simulink model "Flyback_non_ideal_simulation0101"  (R2023b)
settings: Solver=VariableStepAuto  StartTime=0.0  StopTime=0.01  RelTol=1e-3
libraries: spsMeanLib x6, spsCurrentMeasurementLib x4, spsMultimeterLib x4, spsSeriesRLCBranchLib x4, spsDiodeLib x3, spsMosfetLib x3, spsDCVoltageSourceLib x2, spsLinearTransformerLib x2, spsRMSLib x2, spsVoltageMeasurementLib x2, sps_lib x1
settings Model: Creator=User  LastModifiedBy=ozgur

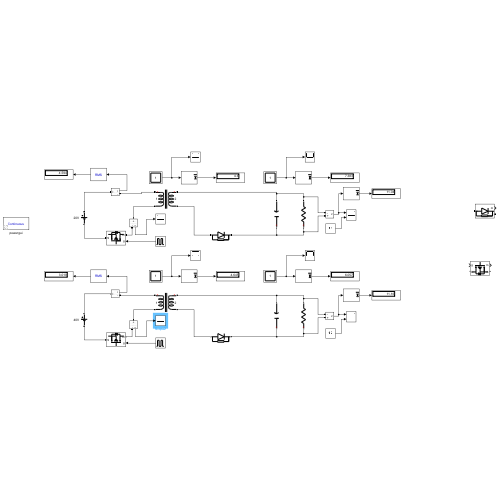
[thumbnail: Simulink's stored preview of the top-level diagram]
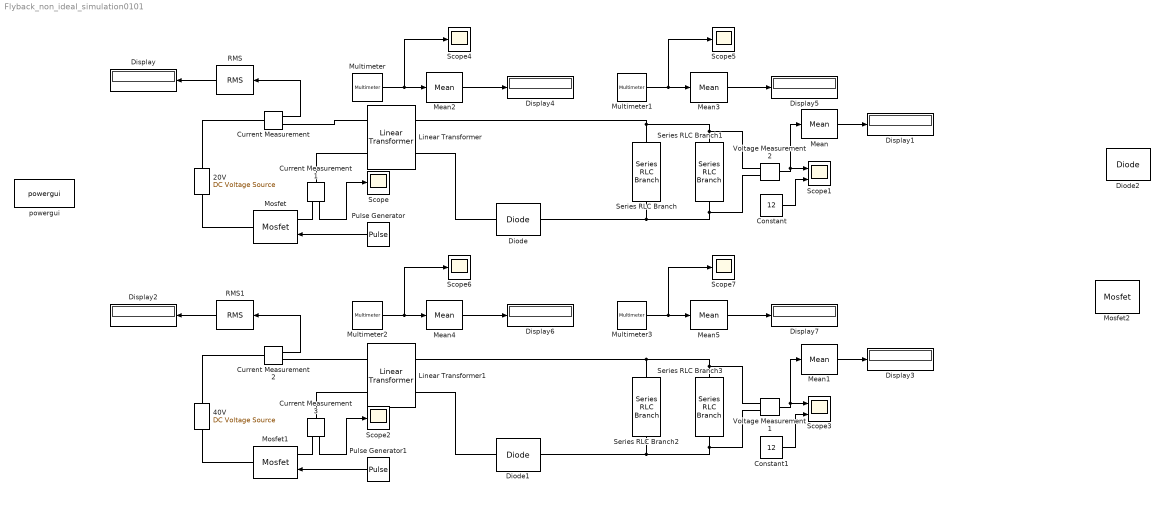
== system Flyback_non_ideal_simulation0101 ==
  20V : spsDCVoltageSourceLib/DC Voltage Source  Amplitude=20  Measurements=None
  40V : spsDCVoltageSourceLib/DC Voltage Source  Amplitude=40  Measurements=None
  Constant : Constant  Value=12
  Constant1 : Constant  Value=12
  Current Measurement{,1..3} (4 alike) : spsCurrentMeasurementLib/Current Measurement  PhasorSimulation=off  OutputType=Complex  PSBequivalent=0
  Diode : spsDiodeLib/Diode  Ron=0.01  Lon=0  Vf=0.65  IC=0  UseSnubber=0  Rs=500  Cs=250e-9  Measurements=off
  Diode1 : spsDiodeLib/Diode  Ron=0  Lon=0  Vf=0.65  IC=0  UseSnubber=0  Rs=500  Cs=250e-9  Measurements=off
  Diode2 : spsDiodeLib/Diode  Ron=0.001  Lon=0  Vf=0.8  IC=0  UseSnubber=0  Rs=500  Cs=250e-9  Measurements=on
  Display{,1..7} (8 alike) : Display
  Linear Transformer : spsLinearTransformerLib/Linear Transformer  UNITS=SI  NominalPower=[ 250 100e3 ]  winding1=[50 0.0042 10e-9]  winding2=[50 0.0042 10e-9]  ThreeWindings=off  winding3=[3.15e+05 7.938e+05 50.535]  RmLm=[1e+05 19.6e-6]  Measurements=All voltages and currents  DataType=on
  Linear Transformer1 : spsLinearTransformerLib/Linear Transformer  UNITS=SI  NominalPower=[ 250 100e3 ]  winding1=[50 0.0042 10e-9]  winding2=[50 0.0042 10e-9]  ThreeWindings=off  winding3=[3.15e+05 7.938e+05 50.535]  RmLm=[1e+05 19.6e-6]  Measurements=All voltages and currents  DataType=on
  Mean{,1..5} (6 alike) : spsMeanLib/Mean  Freq=100e3  Vinit=0  Ts=0
  Mosfet : spsMosfetLib/Mosfet  Ron=44e-3  Lon=0  Rd=0.01  Vfd=0.01  IC=0  Rs=1e5  Cs=inf  Measurements=off
  Mosfet1 : spsMosfetLib/Mosfet  Ron=44e-3  Lon=0  Rd=0.01  Vfd=0.01  IC=0  Rs=1e5  Cs=inf  Measurements=off
  Mosfet2 : spsMosfetLib/Mosfet  Ron=0.1  Lon=0  Rd=0.01  Vfd=0  IC=0  Rs=1e5  Cs=inf  Measurements=on
  Multimeter : spsMultimeterLib/Multimeter  L=14  sel=6  yselected={}  Gain=1  OutputType=Complex  PlotAtSimulationStop=off  PhasorSimulation=off
  Multimeter1 : spsMultimeterLib/Multimeter  L=14  sel=10  yselected={}  Gain=1  OutputType=Complex  PlotAtSimulationStop=off  PhasorSimulation=off
  Multimeter2 : spsMultimeterLib/Multimeter  L=14  sel=8  yselected={}  Gain=1  OutputType=Complex  PlotAtSimulationStop=off  PhasorSimulation=off
  Multimeter3 : spsMultimeterLib/Multimeter  L=14  sel=13  yselected={}  Gain=1  OutputType=Complex  PlotAtSimulationStop=off  PhasorSimulation=off
  Pulse Generator : DiscretePulseGenerator  PulseType=Time based  Period=1/100e3  PulseWidth=37.5
  Pulse Generator1 : DiscretePulseGenerator  PulseType=Time based  Period=1/100e3  PulseWidth=23
  RMS : spsRMSLib/RMS  TrueRMS=on  Freq=100e3  RMSInit=0  Ts=0
  RMS1 : spsRMSLib/RMS  TrueRMS=on  Freq=100e3  RMSInit=0  Ts=0
  Scope{,2,4..7} (6 alike) : Scope
  Scope1 : Scope  NumInputPorts=2
  Scope3 : Scope  NumInputPorts=2
  Series RLC Branch : spsSeriesRLCBranchLib/Series RLC Branch  LConnTagsString=__new0  RConnTagsString=__new0  BranchType=C  Resistance=1  Inductance=1e-3  SetiL0=off  InitialCurrent=0  Capacitance=100e-6  Setx0=off  InitialVoltage=0  Measurements=None
  Series RLC Branch1 : spsSeriesRLCBranchLib/Series RLC Branch  LConnTagsString=__new0  RConnTagsString=__new0  BranchType=R  Resistance=2.4  Inductance=1e-3  SetiL0=off  InitialCurrent=0  Capacitance=100e-6  Setx0=off  InitialVoltage=0  Measurements=None
  Series RLC Branch2 : spsSeriesRLCBranchLib/Series RLC Branch  LConnTagsString=__new0  RConnTagsString=__new0  BranchType=C  Resistance=1  Inductance=1e-3  SetiL0=off  InitialCurrent=0  Capacitance=100e-6  Setx0=off  InitialVoltage=0  Measurements=None
  Series RLC Branch3 : spsSeriesRLCBranchLib/Series RLC Branch  LConnTagsString=__new0  RConnTagsString=__new0  BranchType=R  Resistance=2.4  Inductance=1e-3  SetiL0=off  InitialCurrent=0  Capacitance=100e-6  Setx0=off  InitialVoltage=0  Measurements=None
  Voltage Measurement1 : spsVoltageMeasurementLib/Voltage Measurement  PhasorSimulation=off  OutputType=Complex  PSBequivalent=0
  Voltage Measurement2 : spsVoltageMeasurementLib/Voltage Measurement  PhasorSimulation=off  OutputType=Complex  PSBequivalent=0
  powergui : sps_lib/powergui  Priority=1  SimulationMode=Continuous  SampleTime=50e-6  frequency=60  Iterations=50  frequencyindice=0  Pbase=100e6  ErrMax=1e-4  UnitsV=kV  UnitsW=MW  buscounter=0  FunctionMessages=off  echomessages=off  EnableUseOfTLC=off  CurrentSourceSwitches=off  DisableSnubberDevices=off  DisableRonSwitches=off  DisableVfSwitches=off  DisplayEquations=off  AutomaticDiscreteSolvers=off  SolverType=Tustin/Backward Euler (TBE)  Interpol=off  ExternalGateDelay=off  methode=off  Ts=100  x0status=blocks  SPID=on  SwTol=0  HookPort=off  NonlinearTolerance=1e-4  nMaxIteration=100  ContinueOnMaxIteration=off  RestoreLinks=warning  ResistiveCurrentMeasurement=off  Frange=[0:2:500]  Ylog=off  Xlog=on  ShowGrid=off  save=off  variable=ZData  structure=0  ZoomFFT=off  StartTime=0.0  cycles=1  DisplayStyle=1  fundamental=60  FreqAxis=off  MaxFrequency=1000  frequencyindicesteady=1  RmsSteady=1  display=off
  wires:
  Current Measurement/1 -> RMS/1
  RMS/1 -> Display/1
  Pulse Generator/1 -> Mosfet/1
  Current Measurement1/1 -> Scope/1
  Voltage Measurement2/1 -> Mean/1, Scope1/1
  Mean/1 -> Display1/1
  Mean1/1 -> Display3/1
  Voltage Measurement1/1 -> Mean1/1, Scope3/1
  Pulse Generator1/1 -> Mosfet1/1
  RMS1/1 -> Display2/1
  Current Measurement3/1 -> Scope2/1
  Current Measurement2/1 -> RMS1/1
  Multimeter/1 -> Mean2/1, Scope4/1
  Mean2/1 -> Display4/1
  Multimeter1/1 -> Mean3/1, Scope5/1
  Mean3/1 -> Display5/1
  Multimeter3/1 -> Mean5/1, Scope7/1
  Mean5/1 -> Display7/1
  Multimeter2/1 -> Mean4/1, Scope6/1
  Mean4/1 -> Display6/1
  Constant/1 -> Scope1/2
  Constant1/1 -> Scope3/2
  connections:
  Mosfet/RConn1 -- 20V/LConn1
  20V/RConn1 -- Current Measurement/LConn1
  Current Measurement/RConn1 -- Linear Transformer/LConn1
  Linear Transformer/LConn2 -- Current Measurement1/LConn1
  Current Measurement1/RConn1 -- Mosfet/LConn1
  Linear Transformer/RConn2 -- Diode/LConn1
  Diode/RConn1 -- Series RLC Branch/LConn1 -- Voltage Measurement2/LConn1 -- Series RLC Branch1/LConn1
  Linear Transformer/RConn1 -- Series RLC Branch/RConn1 -- Voltage Measurement2/LConn2 -- Series RLC Branch1/RConn1
  Series RLC Branch3/RConn1 -- Voltage Measurement1/LConn2 -- Series RLC Branch2/RConn1 -- Linear Transformer1/RConn1
  Diode1/RConn1 -- Series RLC Branch2/LConn1 -- Voltage Measurement1/LConn1 -- Series RLC Branch3/LConn1
  Linear Transformer1/RConn2 -- Diode1/LConn1
  Linear Transformer1/LConn2 -- Current Measurement3/LConn1
  Current Measurement2/RConn1 -- Linear Transformer1/LConn1
  40V/RConn1 -- Current Measurement2/LConn1
  Mosfet1/RConn1 -- 40V/LConn1
  Current Measurement3/RConn1 -- Mosfet1/LConn1
